simulink model "dsp"  (R2018b)
settings: Solver=VariableStepAuto  StartTime=0.0  StopTime=10.0  MaxStep=0.001  RelTol=1e-3
settings Model: Creator=ajay  LastModifiedBy=ajay

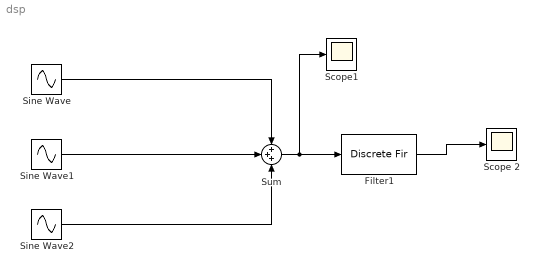
== system dsp ==
  Filter1 : DiscreteFir  Tag=BlockMethodSubSystem  Coefficients=[-0.000898005868309046632 0.00125015489517941092 0.00707870919738830609 0.00919092505074133037 -8.36385587740977864e-18 -0.0145931644543754215 -0.0180072977666334531 -0.00519578938154223804 0.00630801904911239535 -5.14256616555505531e-18 -0.00921081179749107769 0.0111446320670729564 0.0574601580801296363 0.0707325212439469247 -2.11926545896408696e-17 -0.115050612139229125 -0.157744850639242457 -0.0569756631742409023 0.115308309975209342 0.200225548283612165 0.115308309975209342 -0.0569756631742409023 -0.157744850639242457 -0.115050612139229125 -2.11926545896408696e-17 0.0707325212439469247 0.0574601580801296363 0.0111446320670729564 -0.00921081179749107769 -5.14256616555505531e-18 0.00630801904911239535 -0.00519578938154223804 -0.0180072977666334531 -0.0145931644543754215 -8.36385587740977864e-18 0.00919092505074133037 0.00707870919738830609 0.00125015489517941092 -0.000898005868309046632]  InputProcessing=Columns as channels (frame based)
  Scope 2 : Scope
  Scope1 : Scope
  Sine Wave : Sin  Frequency=2*pi*5  SampleTime=0
  Sine Wave1 : Sin  Frequency=2*pi*15  SampleTime=0
  Sine Wave2 : Sin  Frequency=2*pi*30  SampleTime=0
  Sum : Sum  Inputs=+++
  wires:
  Sine Wave/1 -> Sum/1
  Sine Wave1/1 -> Sum/2
  Sine Wave2/1 -> Sum/3
  Sum/1 -> Scope1/1, Filter1/1
  Filter1/1 -> Scope 2/1
